simulink library "AEMACE8_IN"  (R2021b)
settings: Solver=VariableStepAuto  StartTime=0.0  StopTime=10.0  RelTol=1e-3
values from neighbouring files (symbols this model uses):
  dataAEMACE = 60.0    [applicationDD.sldd]    (also in dataAEMACE.mat = ; dataAEMACE_DD.sldd)
  dataAEMACE8 =     [dataAEMACE8.mat]
settings Model: Creator=ACH  LastModifiedBy=C83127

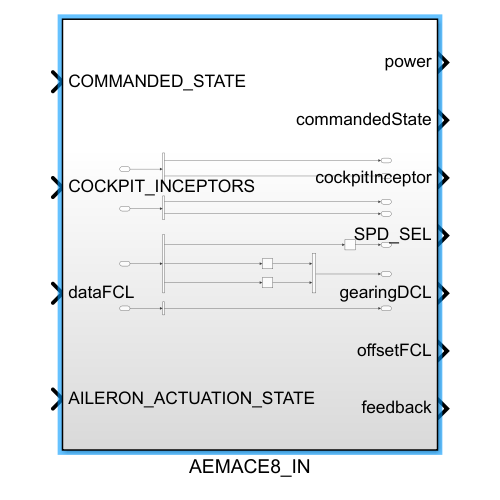
[thumbnail: Simulink's stored preview of the top-level diagram]
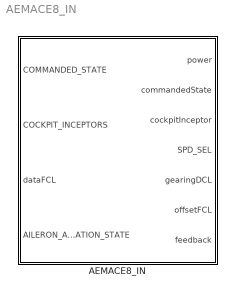
== system AEMACE8_IN ==
  AEMACE8_IN : Subsystem

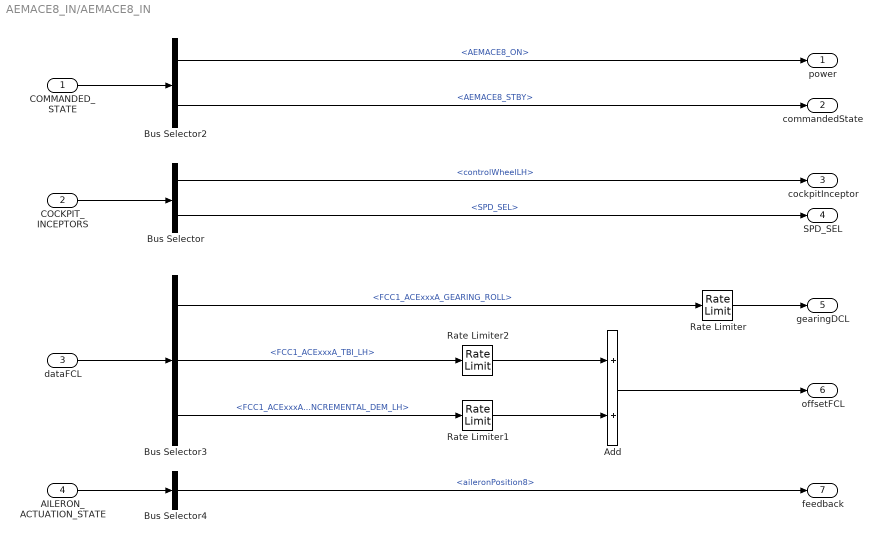
== system AEMACE8_IN/AEMACE8_IN ==
  COMMANDED_STATE : Inport  OutDataTypeStr=Bus: COMMANDED_STATE
  COCKPIT_INCEPTORS : Inport  Port=2  OutDataTypeStr=Bus: COCKPIT_INCEPTORS
  dataFCL : Inport  Port=3  OutDataTypeStr=Bus: FCC1_ACExxxA_C1_A
  AILERON_ACTUATION_STATE : Inport  Port=4  OutDataTypeStr=Bus: AILERON_ACTUATION_STATE
  Add : Sum
  Bus Selector : BusSelector  OutputSignals=controlWheelLH,SPD_SEL
  Bus Selector2 : BusSelector  OutputSignals=AEMACE8_ON,AEMACE8_STBY
  Bus Selector3 : BusSelector  OutputSignals=FCC1_ACExxxA_GEARING_ROLL,FCC1_ACExxxA_TBI_LH,FCC1_ACExxxA_ROLL_INCREMENTAL_DEM_LH
  Bus Selector4 : BusSelector  OutputSignals=aileronPosition8
  Rate Limiter : RateLimiter  RisingSlewLimit=dataAEMACE8.rateLimiterGearing  FallingSlewLimit=-dataAEMACE8.rateLimiterGearing  SampleTimeMode=inherited
      settings: AttributesFormatString=|
      | %<RisingSlewLimit>
      | %<FallingSlewLimit>
  Rate Limiter1 : RateLimiter  RisingSlewLimit=dataAEMACE.rateLimiterIncrementalDemand  FallingSlewLimit=-dataAEMACE.rateLimiterIncrementalDemand  SampleTimeMode=inherited
      settings: AttributesFormatString=|
      | %<RisingSlewLimit>
      | %<FallingSlewLimit>
  Rate Limiter2 : RateLimiter  RisingSlewLimit=dataAEMACE.rateLimiterTBI  FallingSlewLimit=-dataAEMACE.rateLimiterTBI  SampleTimeMode=inherited
      settings: AttributesFormatString=|
      | %<RisingSlewLimit>
      | %<FallingSlewLimit>
  power : Outport
  commandedState : Outport  Port=2
  cockpitInceptor : Outport  Port=3
  SPD_SEL : Outport  Port=4
  gearingDCL : Outport  Port=5
  offsetFCL : Outport  Port=6
  feedback : Outport  Port=7
  wires:
  Bus Selector3/3 -> Rate Limiter1/1  "<FCC1_ACExxxA_ROLL_INCREMENTAL_DEM_LH>"
  Bus Selector3/2 -> Rate Limiter2/1  "<FCC1_ACExxxA_TBI_LH>"
  AILERON_ACTUATION_STATE/1 -> Bus Selector4/1
  Bus Selector2/1 -> power/1  "<AEMACE8_ON>"
  Bus Selector4/1 -> feedback/1  "<aileronPosition8>"
  COMMANDED_STATE/1 -> Bus Selector2/1
  dataFCL/1 -> Bus Selector3/1
  COCKPIT_INCEPTORS/1 -> Bus Selector/1
  Bus Selector/1 -> cockpitInceptor/1  "<controlWheelLH>"
  Bus Selector3/1 -> Rate Limiter/1  "<FCC1_ACExxxA_GEARING_ROLL>"
  Rate Limiter/1 -> gearingDCL/1
  Add/1 -> offsetFCL/1
  Rate Limiter2/1 -> Add/1
  Rate Limiter1/1 -> Add/2
  Bus Selector2/2 -> commandedState/1  "<AEMACE8_STBY>"
  Bus Selector/2 -> SPD_SEL/1  "<SPD_SEL>"
